simulink model "HVDCMMCInterconnection"  (R2024b)
settings: Solver=FixedStepDiscrete  StartTime=0.0  StopTime=11  RelTol=1e-3
PreLoadFcn:
  | GFLParameters_400Kv
  | HVDCMMCInterconnectionParam
StartFcn:
  | tic
StopFcn:
  | toc
values from neighbouring files (symbols this model uses):
  C_PM = 1.758e-3    (= 0.001758)    [HVDCMMCInterconnectionParam.m]
  Cfilter = 1/(Larm*wc2)    (= 4.78421193241e-05)    [HVDCMMCInterconnectionParam.m]
  Cg = 50e-9    (= 5e-08)    [HVDCMMCInterconnectionParam.m]
  Fc = Fnom*3.37    (= 168.5)    [HVDCMMCInterconnectionParam.m]
  Fnom = 50    [GFLParameters_400Kv.m]    (also in HVDCMMCInterconnectionParam.m)
  L_cable = 15e-3    (= 0.015)    [HVDCMMCInterconnectionParam.m]
  Larm = Larm_pu*(Zbase/(2*pi*Fnom))    (= 0.0529455974536)    [HVDCMMCInterconnectionParam.m]
  Limits_Qreg = [ 0.25, -0.25 ]    [HVDCMMCInterconnectionParam.m]
  Lxfo = 0.12    [HVDCMMCInterconnectionParam.m]
  Nb_PM = 36    [HVDCMMCInterconnectionParam.m]
  Pnom = 1000e6    (= 1000000000)    [HVDCMMCInterconnectionParam.m]
  Psc = Pnom*20    (= 20000000000)    [HVDCMMCInterconnectionParam.m]    (also in HVDCMMC_RunFaultAnalysis.m = gridSCLArray(k))
  R_cable = 0.5    [HVDCMMCInterconnectionParam.m]
  R_startup = 400    [HVDCMMCInterconnectionParam.m]
  Rarm = Rarm_pu*Zbase    (= 0.1663335)    [HVDCMMCInterconnectionParam.m]
  Rfilter = 1/(Cfilter*w)*30    (= 1996.002)    [HVDCMMCInterconnectionParam.m]
  Rg = 100    [HVDCMMCInterconnectionParam.m]
  Rxfo = 0.003    [HVDCMMCInterconnectionParam.m]
  Slope_Pref = 0.5    [HVDCMMCInterconnectionParam.m]
  Slope_Qref = 0.5    [HVDCMMCInterconnectionParam.m]
  Slope_Vdc_ref = Vnom_dc/5    (= 128000)    [HVDCMMCInterconnectionParam.m]
  Tbrk1_On = 0.1    [HVDCMMCInterconnectionParam.m]
  Tbrk2_On = 1.0    (= 1)    [HVDCMMCInterconnectionParam.m]
  Tdeblock = 1.5    [HVDCMMCInterconnectionParam.m]
  Tfault = 9999    [HVDCMMCInterconnectionParam.m]
  Ton_Converter2 = 4    [HVDCMMCInterconnectionParam.m]
  Ton_PQreg = 4    [HVDCMMCInterconnectionParam.m]
  Ton_VDCreg = 1.5    [HVDCMMCInterconnectionParam.m]
  Ts = Ts_Control    (= 4e-05)    [HVDCMMCInterconnectionParam.m]
  Ts_Power = 20e-6    (= 2e-05)    [HVDCMMCInterconnectionParam.m]
  Vnom_dc = 640e3    (= 640000)    [HVDCMMCInterconnectionParam.m]
  Vnom_prim = 400e3    (= 400000)    [HVDCMMCInterconnectionParam.m]
  Vnom_sec = 333e3    (= 333000)    [HVDCMMCInterconnectionParam.m]
undefined symbols (not defined in the file or in its folder): ConvCtrl, ConvPlt, DiscIntNeverNeededParam, Discrete, ee_sli_rtmsupport, Fault, gcbh, gridInverter, magnitude, Pcc, PlantSim, sps, sps_rtmsupport, spsPLL3phModel, TL, Trf
libraries: powerlib_extras x27, spsSeriesRLCBranchLib x27, simulink x14, eeGeneralControl x11, spsCurrentMeasurementLib x11, spsVoltageMeasurementLib x8, spsBreakerLib x7, eeTransforms x6, spsHalfBridgeMMCLib x6, spsSecondOrderFilterLib x4, spsabctodq0Lib x4, spsThreePhaseVIMeasurementLib x4
(part 6 of 6)

== system HVDCMMCInterconnection/Controllers/Controllers/Grid-Forming Converter Control/Grid Voltage Reactive Power Support/Modifying Reactive Power Reference/Changing the Power Reference/Estimate Id for Given Iq ==
  Iq : Inport
  Add Constant1 : Bias  Bias=1  SaturateOnIntegerOverflow=off
  Gain : Gain  Gain=-1
  Gain3 : Gain  Gain=0.9
  Sqrt : Sqrt
  Square : Math  Operator=square
  Id : Outport
  wires:
  Square/1 -> Gain/1
  Gain3/1 -> Id/1
  Gain/1 -> Add Constant1/1
  Sqrt/1 -> Gain3/1
  Add Constant1/1 -> Sqrt/1
  Iq/1 -> Square/1

== system HVDCMMCInterconnection/Controllers/Controllers/Grid-Forming Converter Control/Grid Voltage Reactive Power Support/Modifying Reactive Power Reference/Changing the Power Reference/EstimateIqForReactivePower ==
  note: Computing minimum reactive current as per GC0137
  Vmin : Inport
  Vd : Inport  Port=2
  Vs : Inport  Port=3
  Abs : Abs  SaturateOnIntegerOverflow=off
  Add : Sum
  Add Constant : Bias  Bias=1  SaturateOnIntegerOverflow=off
  GC0137 line slope : Gain  Gain=-1.4578
  Low Voltage Support : Subsystem
  Saturation : Saturate  UpperLimit=1  LowerLimit=0
  Iq : Outport
  wires:
  Abs/1 -> GC0137 line slope/1
  GC0137 line slope/1 -> Add Constant/1
  Vs/1 -> Abs/1
  Add/1 -> Saturation/1
  Saturation/1 -> Iq/1
  Add Constant/1 -> Add/2
  Vmin/1 -> Low Voltage Support/1(Vin)
  Vd/1 -> Low Voltage Support/2(Vd)
  Low Voltage Support/1(Iqsupport) -> Add/1

== system HVDCMMCInterconnection/Controllers/Controllers/Grid-Forming Converter Control/Grid Voltage Reactive Power Support/Modifying Reactive Power Reference/Changing the Power Reference/ReactivePowerReference ==
  Vd : Inport
  Iq : Inport  Port=2
  Compute Power : Product
  Constant : Constant  Value=0.3
  Gain2 : Gain  Gain=1.05
  Switch : Switch  Criteria=u2 > Threshold  Threshold=0.3  SaturateOnIntegerOverflow=off  InputSameDT=off
  QrefNew : Outport
  wires:
  Compute Power/1 -> QrefNew/1
  Gain2/1 -> Compute Power/2
  Constant/1 -> Switch/3
  Iq/1 -> Gain2/1
  Vd/1 -> Switch/2, Switch/1
  Switch/1 -> Compute Power/1

== system HVDCMMCInterconnection/Controllers/Controllers/Grid-Forming Converter Control/Measurement/Frequency Measurement/Frequency Measurement/If Action Subsystem ==
  V : Inport
  Time : Inport  Port=2
  Action Port : ActionPort  ActionPortLabel=if(u1 > 0.9)
  Constant1 : Constant  Value=initialFrequency
  Delay : Delay  DelayLength=1
  Delay1 : Delay  DelayLength=1
  Frequency estimation : Subsystem  TreatAsAtomicUnit=on
  Hit Crossing : HitCross
  Switch : Switch  Criteria=u2 > Threshold  Threshold=1  SaturateOnIntegerOverflow=off  InputSameDT=off
  Freq : Outport
  wires:
  V/1 -> Delay/1, Frequency estimation/1(sk), Hit Crossing/1
  Delay1/1 -> Frequency estimation/4(k-1)
  Hit Crossing/1 -> Frequency estimation/Trigger
  Delay/1 -> Frequency estimation/2(sk-1)
  Time/1 -> Switch/2, Delay1/1, Frequency estimation/3(k)
  Frequency estimation/1(f) -> Switch/1
  Constant1/1 -> Switch/3
  Switch/1 -> Freq/1

== system HVDCMMCInterconnection/Controllers/Controllers/Grid-Forming Converter Control/Measurement/Frequency Measurement/Frequency Measurement/If Action Subsystem1 ==
  Action Port : ActionPort  ActionPortLabel=else
  Constant1 : Constant  Value=initialFrequency
  Out1 : Outport
  wires:
  Constant1/1 -> Out1/1

== system HVDCMMCInterconnection/Controllers/Controllers/Grid-Forming Converter Control/Measurement/Frequency Measurement/Frequency Measurement/Postive Sequence ==
  abc : Inport
  Complex to Real-Imag : ComplexToRealImag
  Demux : Demux  Outputs=3
  Symmetrical-Components Transform : eeTransforms/Symmetrical-Components Transform  PowerInvariant=off
      settings: LibrarySourceBlock=|
      | ee_sl_lib/Mathematical
      | Transforms/Symmetrical-Components
      | Transform
  Terminator : Terminator
  Terminator1 : Terminator
  Terminator2 : Terminator
  posSeq : Outport
  wires:
  abc/1 -> Symmetrical-Components Transform/1
  Symmetrical-Components Transform/1 -> Demux/1
  Complex to Real-Imag/1 -> posSeq/1
  Demux/1 -> Complex to Real-Imag/1
  Complex to Real-Imag/2 -> Terminator/1
  Demux/2 -> Terminator1/1
  Demux/3 -> Terminator2/1

== system HVDCMMCInterconnection/Controllers/Controllers/Grid-Forming Converter Control/Measurement/abc2dq/Supply Current to dq/Park Transform ==
  abc : Inport
  theta : Inport  Port=2
  0 : Fcn  Expr=K1*(u(1) + u(2) + u(3))
  Gain1 : Gain  Gain=K2
  Mux2 : Mux  Inputs=2
  Mux3 : Mux  Inputs=3
  d : Fcn  Expr=sin(u(4)+Offset)*u(1) + sin(u(4)+Offset-2*pi/3)*u(2) + sin(u(4)+Offset+2*pi/3)*u(3)
  q : Fcn  Expr=cos(u(4)+Offset)*u(1) + cos(u(4)+Offset-2*pi/3)*u(2) + cos(u(4)+Offset+2*pi/3)*u(3)
  dq0 : Outport  VectorParamsAs1DForOutWhenUnconnected=off
  wires:
  0/1 -> Mux3/3
  Gain1/1 -> dq0/1
  Mux3/1 -> Gain1/1
  theta/1 -> Mux2/2
  q/1 -> Mux3/2
  d/1 -> Mux3/1
  abc/1 -> Mux2/1
  Mux2/1 -> 0/1, q/1, d/1

== system HVDCMMCInterconnection/Controllers/Controllers/Grid-Forming Converter Control/Measurement/abc2dq/Supply Voltage  to dq/Park Transform ==
  abc : Inport
  theta : Inport  Port=2
  0 : Fcn  Expr=K1*(u(1) + u(2) + u(3))
  Gain1 : Gain  Gain=K2
  Mux2 : Mux  Inputs=2
  Mux3 : Mux  Inputs=3
  d : Fcn  Expr=sin(u(4)+Offset)*u(1) + sin(u(4)+Offset-2*pi/3)*u(2) + sin(u(4)+Offset+2*pi/3)*u(3)
  q : Fcn  Expr=cos(u(4)+Offset)*u(1) + cos(u(4)+Offset-2*pi/3)*u(2) + cos(u(4)+Offset+2*pi/3)*u(3)
  dq0 : Outport  VectorParamsAs1DForOutWhenUnconnected=off
  wires:
  0/1 -> Mux3/3
  Gain1/1 -> dq0/1
  Mux3/1 -> Gain1/1
  theta/1 -> Mux2/2
  q/1 -> Mux3/2
  d/1 -> Mux3/1
  abc/1 -> Mux2/1
  Mux2/1 -> 0/1, q/1, d/1

== system HVDCMMCInterconnection/Controllers/Controllers/Grid-Forming Converter Control/Power Control/ActivePowerControl/vsmControl/Damping Frequency ==
  fref : Inport
  ConstantFreqReference : Subsystem  VariantControl=constFreq
  WithFrequencyMeasurement : Subsystem  VariantControl=freqMeas
  fmeas : Outport

== system HVDCMMCInterconnection/Controllers/Controllers/Grid-Following Converter Control/PLL, Measurements and Transformation/PLL (3ph)/Model/Subsystem/Discrete ==
  Err : Inport  SampleTime=Ts
  "Discrete Derivative " : DiscreteTransferFcn  Numerator="[ 1  -1 ]*Kd"  Denominator="[ TcD  Ts-TcD ]"  SampleTime=Ts
  Discrete-Time Integrator : DiscreteIntegrator  gainval=Ki  InitialCondition=Init  SampleTime=Ts  LimitOutput=on  UpperSaturationLimit=Par_Limits(1)  LowerSaturationLimit=Par_Limits(2)  ICPrevOutput=DiscIntNeverNeededParam  ICPrevScaledInput=DiscIntNeverNeededParam
  Kp4 : Gain  Gain=Kp  SaturateOnIntegerOverflow=on  SampleTime=Ts  OutDataTypeStr=Inherit: Same as input  ParamDataTypeStr=Inherit: Same as input
  Saturation1 : Saturate  UpperLimit=Par_Limits(1)  LowerLimit=Par_Limits(2)  SampleTime=Ts
  Sum6 : Sum  Inputs=+++  InputSameDT=on  SaturateOnIntegerOverflow=on  SampleTime=Ts  OutDataTypeStr=Inherit: Same as first input
  Out : Outport  SampleTime=Ts  InitialOutput=0  VectorParamsAs1DForOutWhenUnconnected=off
  wires:
  Saturation1/1 -> Out/1
  Err/1 -> "Discrete Derivative "/1, Discrete-Time Integrator/1, Kp4/1
  Sum6/1 -> Saturation1/1
  Kp4/1 -> Sum6/1
  Discrete-Time Integrator/1 -> Sum6/2
  "Discrete Derivative "/1 -> Sum6/3

== system HVDCMMCInterconnection/Controllers/Controllers/Grid-Forming Converter Control/Current Limiting/CurrentLimitingMethod/currentLimitAndVirtual/Current Saturation/Compare ==
  u : Inport
  Compare To Zero : simulink/Logic and Bit Operations/Compare To Zero  relop=<=  OutDataTypeStr=boolean
  Data Type Conversion : DataTypeConversion  SaturateOnIntegerOverflow=off  RndMeth=Floor
  Out1 : Outport
  wires:
  Compare To Zero/1 -> Data Type Conversion/1
  u/1 -> Compare To Zero/1
  Data Type Conversion/1 -> Out1/1

== system HVDCMMCInterconnection/Controllers/Controllers/Grid-Forming Converter Control/Current Limiting/CurrentLimitingMethod/currentLimitAndVirtual/Current Saturation/If Action Subsystem ==
  Is : Inport
  Isd : Inport  Port=2
  Isq : Inport  Port=3
  maxI : Inport  Port=4
  Action Port : ActionPort
  Divide : Product  Inputs=*/
  Product : Product
  Product1 : Product
  Idmax : Outport
  Iqmax : Outport  Port=2
  wires:
  maxI/1 -> Divide/1
  Is/1 -> Divide/2
  Divide/1 -> Product1/2, Product/1
  Isd/1 -> Product1/1
  Isq/1 -> Product/2
  Product1/1 -> Idmax/1
  Product/1 -> Iqmax/1

== system HVDCMMCInterconnection/Controllers/Controllers/Grid-Forming Converter Control/Current Limiting/CurrentLimitingMethod/currentLimitAndVirtual/Current Saturation/If Action Subsystem1 ==
  Action Port : ActionPort
  Constant3 : Constant  Value=0
  Constant4 : Constant  Value=0
  Idmax : Outport
  Iqmax : Outport  Port=2
  wires:
  Constant4/1 -> Iqmax/1
  Constant3/1 -> Idmax/1

== system HVDCMMCInterconnection/Controllers/Controllers/Grid-Forming Converter Control/Grid Voltage Reactive Power Support/Modifying Reactive Power Reference/Changing the Power Reference/EstimateIqForReactivePower/Low Voltage Support ==
  Vin : Inport
  Vd : Inport  Port=2
  Gain4 : Gain  Gain=lowVoltageSupportGain
  Saturation1 : Saturate  UpperLimit=1  LowerLimit=-1
  Subtract : Sum  Inputs=+-
  Iqsupport : Outport
  wires:
  Subtract/1 -> Gain4/1
  Gain4/1 -> Saturation1/1
  Saturation1/1 -> Iqsupport/1
  Vin/1 -> Subtract/1
  Vd/1 -> Subtract/2

== system HVDCMMCInterconnection/Controllers/Controllers/Grid-Forming Converter Control/Measurement/Frequency Measurement/Frequency Measurement/If Action Subsystem/Frequency estimation ==
  sk : Inport
  sk-1 : Inport  Port=2
  k : Inport  Port=3
  k-1 : Inport  Port=4
  Trigger : TriggerPort  VariantControl=(inherit)  InitialTriggerSignalState=positive
  Add1 : Sum  Inputs=+-  OutDataTypeStr=double  AccumDataTypeStr=double  RndMeth=Convergent
  Add2 : Sum
  Constant : Constant
  Delay : Delay  DelayLength=1
  Delay1 : Delay  DelayLength=1
  Divide : Product  Inputs=*/  RndMeth=Ceiling
  Gain : Gain  Gain=2  ParamDataTypeStr=double  RndMeth=Convergent
  Gain2 : Gain  Gain=0.5
  MATLAB Function : MATLAB Function  TreatAsAtomicUnit=on
  f : Outport
  wires:
  Add1/1 -> Gain/1
  Constant/1 -> Divide/1
  Gain/1 -> Divide/2
  MATLAB Function/1(x) -> Delay/1, Add1/1  "x1-y1/slope"
  Divide/1 -> Add2/1, Delay1/1
  Delay1/1 -> Add2/2
  Add2/1 -> Gain2/1
  Gain2/1 -> f/1
  Delay/1 -> Add1/2
  k/1 -> MATLAB Function/3(x1)
  k-1/1 -> MATLAB Function/4(x2)  "x1"
  sk/1 -> MATLAB Function/1(y1)
  sk-1/1 -> MATLAB Function/2(y2)

== system HVDCMMCInterconnection/Controllers/Controllers/Grid-Forming Converter Control/Power Control/ActivePowerControl/vsmControl/Damping Frequency/ConstantFreqReference ==
  fref : Inport
  Constant1 : Constant
  Terminator : Terminator
  fmeas : Outport
  wires:
  Constant1/1 -> fmeas/1
  fref/1 -> Terminator/1

== system HVDCMMCInterconnection/Controllers/Controllers/Grid-Forming Converter Control/Power Control/ActivePowerControl/vsmControl/Damping Frequency/WithFrequencyMeasurement ==
  fref : Inport
  fmeas : Outport
  wires:
  fref/1 -> fmeas/1

== matlab function HVDCMMCInterconnection/Controllers/Controllers/Grid-Following Converter Control/Mode of Operation Panel/MATLAB Function (Mode of Operation - Converter 1) ==
  data: u input
function fcn(u)
coder.extrinsic('set_param')
coder.extrinsic('evalin')
%#codegen
gcs1='HVDC_MMC';
switch u
    case 1
        set_param([gcs1, '/Mode1'], 'ForegroundColor', 'red')
        set_param([gcs1, '/Mode2'], 'ForegroundColor', '[ 0.808, 0.808, 0.808]')
        set_param([gcs1, '/Mode3'], 'ForegroundColor', '[ 0.808, 0.808, 0.808]')
        set_param([gcs1, '/Brk1'], 'BackgroundColor', 'yellow')
        set_param([gcs1, '/Brk2'], 'BackgroundColor', 'white')
        set_param([gcs1, '/R_startup'], 'BackgroundColor', 'yellow')
        set_param([gcs1, '/Tr1'], 'BackgroundColor', 'yellow')
        set_param([gcs1, '/Ld2'], 'BackgroundColor', 'yellow')
        set_param([gcs1, '/Half-Bridge MMC Ap'], 'BackgroundColor', 'yellow')
        set_param([gcs1, '/Half-Bridge MMC Bp'], 'BackgroundColor', 'yellow')
        set_param([gcs1, '/Half-Bridge MMC Cp'], 'BackgroundColor', 'yellow')
        set_param([gcs1, '/Half-Bridge MMC Am'], 'BackgroundColor', 'yellow')
        set_param([gcs1, '/Half-Bridge MMC Bm'], 'BackgroundColor', 'yellow')
        set_param([gcs1, '/Half-Bridge MMC Cm'], 'BackgroundColor', 'yellow') 
        evalin('base','soundsc(Y,FS)')
    case 2
        set_param([gcs1, '/Brk2'], 'BackgroundColor', 'yellow')
        set_param([gcs1, '/R_startup'], 'BackgroundColor', 'white')
        evalin('base','soundsc(Y,FS)')
    case 3
        set_param([gcs1, '/Mode1'], 'ForegroundColor', '[ 0.808, 0.808, 0.808]')
        set_param([gcs1, '/Mode2'], 'ForegroundColor', 'red')
        set_param([gcs1, '/Mode3'], 'ForegroundColor', '[ 0.808, 0.808, 0.808]')
        evalin('base','soundsc(Y,FS)')
    case 4
        set_param([gcs1, '/Mode1'], 'ForegroundColor', '[ 0.808, 0.808, 0.808]')
        set_param([gcs1, '/Mode2'], 'ForegroundColor', '[ 0.808, 0.808, 0.808]')
        set_param([gcs1, '/Mode3'], 'ForegroundColor', 'red')
        evalin('base','soundsc(Y,FS)')
    otherwise
        set_param([gcs1, '/Mode1'], 'ForegroundColor', '[ 0.808, 0.808, 0.808]')
        set_param([gcs1, '/Mode2'], 'ForegroundColor', '[ 0.808, 0.808, 0.808]')
        set_param([gcs1, '/Mode3'], 'ForegroundColor', '[ 0.808, 0.808, 0.808]')
        set_param([gcs1, '/400-kV Equivalent'], 'BackgroundColor', 'yellow')
        set_param([gcs1, '/Ld1'], 'BackgroundColor', 'yellow')
        set_param([gcs1, '/R_startup'], 'BackgroundColor', 'white')
        set_param([gcs1, '/Brk1'], 'BackgroundColor', 'white')
        set_param([gcs1, '/Brk2'], 'BackgroundColor', 'white')
        set_param([gcs1, '/Tr1'], 'BackgroundColor', 'white')
        set_param([gcs1, '/Ld2'], 'BackgroundColor', 'white')
        set_param([gcs1, '/Half-Bridge MMC Ap'], 'BackgroundColor', 'white')
        set_param([gcs1, '/Half-Bridge MMC Bp'], 'BackgroundColor', 'white')
        set_param([gcs1, '/Half-Bridge MMC Cp'], 'BackgroundColor', 'white')
        set_param([gcs1, '/Half-Bridge MMC Am'], 'BackgroundColor', 'white')
        set_param([gcs1, '/Half-Bridge MMC Bm'], 'BackgroundColor', 'white')
        set_param([gcs1, '/Half-Bridge MMC Cm'], 'BackgroundColor', 'white')
end

== stateflow chart HVDCMMCInterconnection/Controllers/Controllers/Grid-Forming Converter Control/Current Limiting/CurrentLimitingMethod/currentLimitAndVirtual/CurrentLimitSelection ==
  state Mode1_VI_ON
    entry:
    noCurrentLimit  = 0;
    viCurrentLimit = 1;
    satCurrentLimit = 0;
    ismax= maxVICurrentLimit;
    exit:
    noCurrentLimit  = 0;
    viCurrentLimit = 1;
    satCurrentLimit = 0;
    ismax= maxVICurrentLimit;
  state Start_Mode
    entry:
    noCurrentLimit  = 1;
    viCurrentLimit = 0;
    satCurrentLimit = 0;
    ismax= maxSatCurrentLimit;
    exit:
    noCurrentLimit  = 1;
    viCurrentLimit = 0;
    satCurrentLimit = 0;
    ismax= maxSatCurrentLimit;
  state Mode2_CurrentSat_ON
    entry:
    noCurrentLimit  = 0;
    viCurrentLimit = 0;
    satCurrentLimit = 1;
    ismax= maxSatCurrentLimit;
    exit:
    noCurrentLimit  = 0;
    viCurrentLimit = 0;
    satCurrentLimit = 1;
    ismax= maxSatCurrentLimit;
  state Mode3_CurrentSat_ON
    entry:
    noCurrentLimit  = 0;
    viCurrentLimit = 0;
    satCurrentLimit = 1;
    ismax= maxVICurrentLimit;
    exit:
    noCurrentLimit  = 0;
    viCurrentLimit = 0;
    satCurrentLimit = 1;
    ismax= 0.97*maxVICurrentLimit;
  Start_Mode -> Mode1_VI_ON : [Is>1]
  (junction 28) -> Mode1_VI_ON : after(modeTransferTime, sec)[(Is<ismax) && (Is>1) ]
  Mode3_CurrentSat_ON -> (junction 28) [order 1]
  (default) -> Start_Mode
  Mode1_VI_ON -> Start_Mode [order 2] : [Is<1]
  Mode1_VI_ON -> Mode2_CurrentSat_ON [order 1] : after(1/powerFreq, sec)[(Is>=maxSatCurrentLimit)]
  (junction 26) -> Start_Mode
  Mode2_CurrentSat_ON -> Mode3_CurrentSat_ON : after(currentSatTime, sec)[satCurrentLimit>0]
  Mode3_CurrentSat_ON -> (junction 26) [order 2] : [Is<1]
  data: Is input; ismax output; noCurrentLimit output; viCurrentLimit output; satCurrentLimit output; maxSatCurrentLimit parameter; maxVICurrentLimit parameter; currentSatTime parameter; powerFreq parameter; modeTransferTime parameter

== matlab function HVDCMMCInterconnection/Controllers/Controllers/Grid-Forming Converter Control/Measurement/Frequency Measurement/Frequency Measurement/If Action Subsystem/Frequency estimation/MATLAB Function ==
  data: y1 input; y2 input; x1 input; x output; x2 input
function x = fcn(y1,y2,x1,x2)
% Line equation between two points is y-y1=((y2-y1)/(x2-x1))*(x-x1). Here
% to to find the zero crossing instant substitute y = 0 and find x
slope = (y2-y1)/(x2-x1);
x = x1-y1/slope;
